simulink model "SystemARMAX_2"  (Simulink 10.2)
settings: Solver=FixedStepDiscrete  StartTime=0.0  StopTime=tend  RelTol=1e-3  EnableMultiTasking=on
values from neighbouring files (symbols this model uses):
  c1o = 0    [zad_1_1.m]    (also in zad_1_2.m = 0.99; zad_2_RIV.m = 0.7; zad_2_RLS.m)
  ident_select = 0    [zad_1_2.m]    (also in zad_2_RIV.m; zad_2_RLS.m = 1)
  Td = 1500    [zad_1_1.m]    (also in zad_1_2.m; zad_2_RIV.m = 500; zad_2_RLS.m = 500)
  Tp = 0.1    [zad_1_1.m]    (also in zad_1_2.m; zad_2_RIV.m; zad_2_RLS.m)
libraries: simulink x2
settings Model: Creator=anraf1001  LastModifiedBy=anraf1001
settings DataIOCC: LimitDataPoints=on
settings OptimizationCC: InitFltsAndDblsToZero=on
settings DebuggingCC: SaveWithParameterizedLinksMsg=none  SignalResolutionControl=TryResolveAllWithWarning  SolverPrmCheckMsg=warning  MultiTaskDSMMsg=warning  MultiTaskCondExecSysMsg=none
settings SFSimCC: SimUseLocalCustomCode=on  CustomCodeUndefinedFunction=FilterOut
settings RTWCC: RTWUseLocalCustomCode=on
settings GRTTargetCC: TargetFcnLib=ansi_tfl_tmw.mat
settings ConfigComp: CovExternalEMLEnable=on

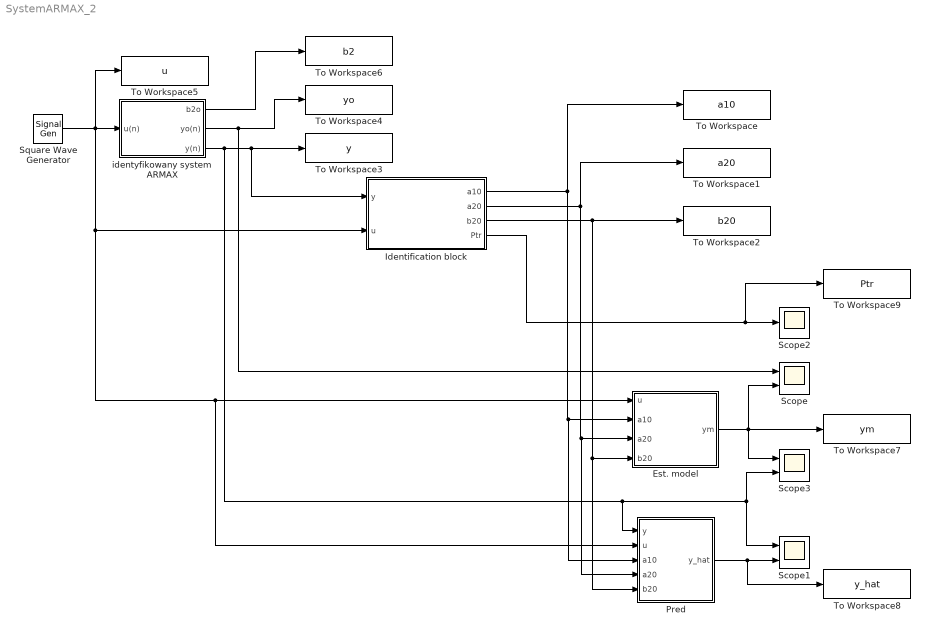
== system SystemARMAX_2 ==
  Est. model : MATLAB Function  TreatAsAtomicUnit=on
  Identification block : Subsystem
  Pred : MATLAB Function  TreatAsAtomicUnit=on
  Scope : Scope  NumInputPorts=2
  Scope1 : Scope  NumInputPorts=2
  Scope2 : Scope
  Scope3 : Scope  NumInputPorts=2
  Square Wave Generator : SignalGenerator  WaveForm=square  Frequency=0.025  Units=rad/sec
  To Workspace : ToWorkspace  VariableName=a10  SampleTime=-1
  To Workspace1 : ToWorkspace  VariableName=a20  SampleTime=-1
  To Workspace2 : ToWorkspace  VariableName=b20  SampleTime=-1
  To Workspace3 : ToWorkspace  VariableName=y  SampleTime=-1
  To Workspace4 : ToWorkspace  VariableName=yo  SampleTime=-1
  To Workspace5 : ToWorkspace  VariableName=u  SampleTime=-1
  To Workspace6 : ToWorkspace  VariableName=b2  SampleTime=-1
  To Workspace7 : ToWorkspace  VariableName=ym  SampleTime=-1
  To Workspace8 : ToWorkspace  VariableName=y_hat  SampleTime=-1
  To Workspace9 : ToWorkspace  VariableName=Ptr  SampleTime=-1
  identyfikowany system ARMAX : Subsystem
  wires:
  Square Wave Generator/1 -> identyfikowany system ARMAX/1(u(n)), To Workspace5/1, Est. model/1(u), Pred/2(u), Identification block/2(u)
  identyfikowany system ARMAX/2(yo(n)) -> To Workspace4/1, Scope/1
  identyfikowany system ARMAX/1(b2o) -> To Workspace6/1
  Est. model/1(ym) -> To Workspace7/1, Scope3/1, Scope/2
  Pred/1(y_hat) -> To Workspace8/1, Scope1/2
  identyfikowany system ARMAX/3(y(n)) -> Identification block/1(y), To Workspace3/1, Pred/1(y), Scope3/2, Scope1/1
  Identification block/4(Ptr) -> To Workspace9/1, Scope2/1
  Identification block/3(b20) -> Pred/5(b20), Est. model/4(b20), To Workspace2/1
  Identification block/2(a20) -> To Workspace1/1, Pred/4(a20), Est. model/3(a20)
  Identification block/1(a10) -> To Workspace/1, Pred/3(a10), Est. model/2(a10)

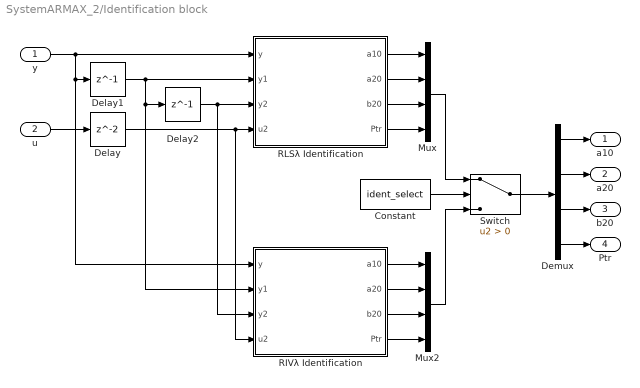
== system SystemARMAX_2/Identification block ==
  y : Inport
  u : Inport  Port=2
  Constant : Constant  Value=ident_select  SampleTime=-1
  Delay : Delay  InitialCondition=0
  Delay1 : Delay  DelayLength=1  InitialCondition=0
  Delay2 : Delay  DelayLength=1  InitialCondition=0
  Demux : Demux
  Mux : Mux
  Mux2 : Mux
  RIVλ Identification : MATLAB Function  TreatAsAtomicUnit=on
  RLSλ Identification : MATLAB Function  TreatAsAtomicUnit=on
  Switch : Switch  Criteria=u2 > Threshold
  a10 : Outport
  a20 : Outport  Port=2
  b20 : Outport  Port=3
  Ptr : Outport  Port=4
  wires:
  Delay2/1 -> RLSλ Identification/3(y2), RIVλ Identification/3(y2)
  y/1 -> RIVλ Identification/1(y), Delay1/1, RLSλ Identification/1(y)
  u/1 -> Delay/1
  Delay/1 -> RIVλ Identification/4(u2), RLSλ Identification/4(u2)
  Delay1/1 -> RLSλ Identification/2(y1), RIVλ Identification/2(y1), Delay2/1
  RLSλ Identification/1(a10) -> Mux/1
  RLSλ Identification/2(a20) -> Mux/2
  RLSλ Identification/3(b20) -> Mux/3
  RLSλ Identification/4(Ptr) -> Mux/4
  RIVλ Identification/1(a10) -> Mux2/1
  RIVλ Identification/2(a20) -> Mux2/2
  RIVλ Identification/3(b20) -> Mux2/3
  RIVλ Identification/4(Ptr) -> Mux2/4
  Mux/1 -> Switch/1
  Mux2/1 -> Switch/3
  Switch/1 -> Demux/1
  Demux/1 -> a10/1
  Demux/2 -> a20/1
  Demux/3 -> b20/1
  Demux/4 -> Ptr/1
  Constant/1 -> Switch/2

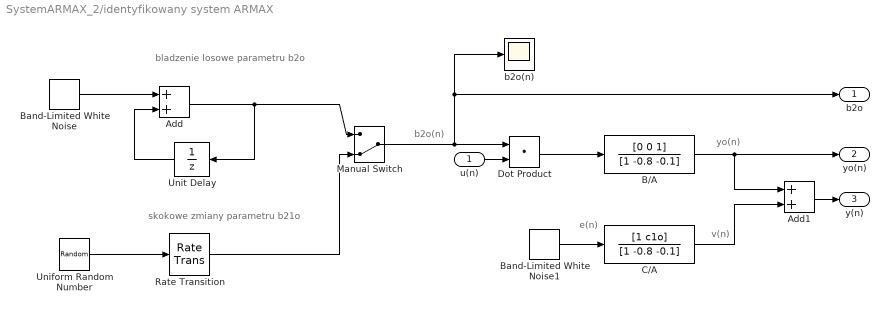
== system SystemARMAX_2/identyfikowany system ARMAX ==
  note: e(n)
  note: v(n)
  note: yo(n)
  note: b2o(n)
  note: skokowe zmiany parametru b21o
  note: bladzenie losowe parametru b2o
  u(n) : Inport
  Add : Sum
  Add1 : Sum
  B/A : DiscreteFilter  Numerator=[0 0 1]  Denominator=[1 -0.8 -0.1]  SampleTime=Tp
  Band-Limited White Noise : simulink/Sources/Band-Limited White Noise  Cov=[0.00001*Tp]  Ts=Tp  seed=[23341]
  Band-Limited White Noise1 : simulink/Sources/Band-Limited White Noise  Cov=[0.001*Tp]  Ts=Tp  seed=[23341]
  C/A : DiscreteFilter  Numerator=[1 c1o]  Denominator=[1 -0.8 -0.1]  SampleTime=Tp
  Dot Product : DotProduct  InputSameDT=on  OutDataTypeStr=Inherit: Inherit via internal rule
  Manual Switch : ManualSwitch  CurrentSetting=0
  Rate Transition : RateTransition  InitialCondition=0.5  OutPortSampleTime=Tp
  Uniform Random Number : UniformRandomNumber  Minimum=0.1  Maximum=0.8  Seed=2  SampleTime=Td
  Unit Delay : UnitDelay  SampleTime=Tp
  b2o(n) : Scope
  b2o : Outport
  yo(n) : Outport  Port=2
  y(n) : Outport  Port=3
  wires:
  Band-Limited White Noise/1 -> Add/1
  Add/1 -> Unit Delay/1, Manual Switch/1
  Unit Delay/1 -> Add/2
  Uniform Random Number/1 -> Rate Transition/1
  Rate Transition/1 -> Manual Switch/2
  Manual Switch/1 -> Dot Product/1, b2o/1, b2o(n)/1
  Dot Product/1 -> B/A/1
  C/A/1 -> Add1/2
  B/A/1 -> Add1/1, yo(n)/1
  Band-Limited White Noise1/1 -> C/A/1
  u(n)/1 -> Dot Product/2
  Add1/1 -> y(n)/1

== matlab function Est. model ==
  data: u input double; ym output double; a10 input double; a20 input double; b20 input double
function ym = fcn(u, a10, a20, b20)
persistent y1
if isempty(y1)
    y1 = 0;
end

persistent y2
if isempty(y2)
    y2 = 0;
end

persistent u1
if isempty(u1)
    u1 = 0;
end

persistent u2
if isempty(u2)
    u2 = 0;
end


ym = -a10 * y1 - a20 * y2 + b20 * u2;

u2 = u1;
u1 = u;

y2 = y1;
y1 = ym;

== matlab function Identification block/RLSλ Identification ==
  data: y input double; y1 input double; y2 input double; a10 output double; u2 input double; a20 output double; b20 output double; Ptr output double
function [a10, a20, b20, Ptr] = fcn(y, y1, y2, u2)
persistent p
if isempty(p)
    p = zeros(3, 1);
end

persistent P
if isempty(P)
%     P = eye(3);
    P = [10, 0, 0; 0, 1, 0; 0, 0, 0.1];
end

lambda = 0.98;

phi = [-y1; -y2; u2];
P = 1/lambda * (P - (P * (phi * phi') * P) / (1 + phi' * P * phi));
k = P * phi;
e = y - phi' * p;
p = p + k * e;

a10 = p(1);
a20 = p(2);
b20 = p(3);
Ptr = trace(P);

== matlab function Pred ==
  data: y input double; u input double; y_hat output double; a10 input double; a20 input double; b20 input double
function y_hat = fcn(y, u, a10, a20, b20)
persistent y1
if isempty(y1)
    y1 = 0;
end

persistent y2
if isempty(y2)
    y2 = 0;
end

persistent u1
if isempty(u1)
    u1 = 0;
end

persistent u2
if isempty(u2)
    u2 = 0;
end


y_hat = -a10 * y1 - a20 * y2 + b20 * u2;

u2 = u1;
u1 = u;

y2 = y1;
y1 = y;

== matlab function Identification block/RIVλ Identification ==
  data: y input double; y1 input double; y2 input double; a10 output double; u2 input double; a20 output double; b20 output double; Ptr output double
function [a10, a20, b20, Ptr] = fcn(y, y1, y2, u2)
persistent p
if isempty(p)
    p = zeros(3, 1);
end

persistent P
if isempty(P)
%     P = eye(3);
    P = [10, 0, 0; 0, 1, 0; 0, 0, 0.1];
end

persistent z
if isempty(z)
    z = zeros(3, 1);
end

z(3) = u2;
phi = [-y1; -y2; u2];
x = z' * p;
P = P - (P * (z * phi') * P) / (1 + phi' * P * z);
k = P * z;
e = y - phi' * p;
p = p + k * e;

z(2) = z(1);
z(1) = -x;

a10 = p(1);
a20 = p(2);
b20 = p(3);
Ptr = trace(P);
